simulink model "ForceControl_Quadruped_vmc"  (R2018b)
settings: Solver=FixedStepAuto  StartTime=0.0  StopTime=2  FixedStep=0.001  RelTol=1e-3  EnableMultiTasking=on
undefined symbols (not defined in the file or in its folder): robot, X, Y, Z
libraries: sm_lib x43, nesl_utility x32, Contact_Forces_Lib x4
(part 1 of 3)
settings Model: Creator=gongs  LastModifiedBy=gongs
settings SolverCC: AlgebraicLoopSolver=LineSearch  AutoInsertRateTranBlk=on
settings DataIOCC: LimitDataPoints=on
settings OptimizationCC: LifeSpan=inf
settings DebuggingCC: AllowSymbolicDim=off  SFUnexpectedBacktrackingDiag=warning  SFNoUnconditionalDefaultTransitionDiag=warning  SFExecutionAtInitializationDiag=none
settings SFSimCC: SimUseLocalCustomCode=off
settings RTWCC: RTWUseLocalCustomCode=off
settings CodeAppCC: StateflowObjectComments=on
settings GRTTargetCC: TargetLangStandard=C89/C90 (ANSI)  GeneratePreprocessorConditionals=Disable all
settings ConfigComp: CovMetricSettings=dw  CovHtmlReporting=on  CovSaveCumulativeToWorkspaceVar=on  CovSaveSingleToWorkspaceVar=on  CovExternalEMLEnable=off  CovSFcnEnable=off
settings SimscapeCC: SimscapeNominalValues="[{\"value\":\"10\",\"unit\":\"V\"},{\"value\":\"1\",\"unit\":\"A\"},{\"value\":\"10\",\"unit\":\"N*m\"},{\"value\":\"10\",\"unit\":\"bar\"},{\"value\":\"100\",\"unit\":\"kJ/kg\"},{\"value\":\"1\",\"unit\":\"kW\"},{\"value\":\"300\",\"unit\":\"K\"},{\"value\":\"100\",\"unit\":\"cm^3/s\"},{\"value\":\"1\",\"unit\":\"kN\"},{\"value\":\"1\",\"unit\":\"g/cm^3\"},{\"value\":\"1\",\"unit\":\"l\"},{\"value\":\"1\",\"unit\":\"cm^2\"},{\"value\":\"60\",\"unit\":\"Hz\"}]"  SimscapeLogType=all  SimscapeLogDataHistory=10000
settings ConfigurationSet: Description=SimMechanics 2G
settings DiagnosticsConfigSet: SimMechanicsRigidlyBoundBlock=warning

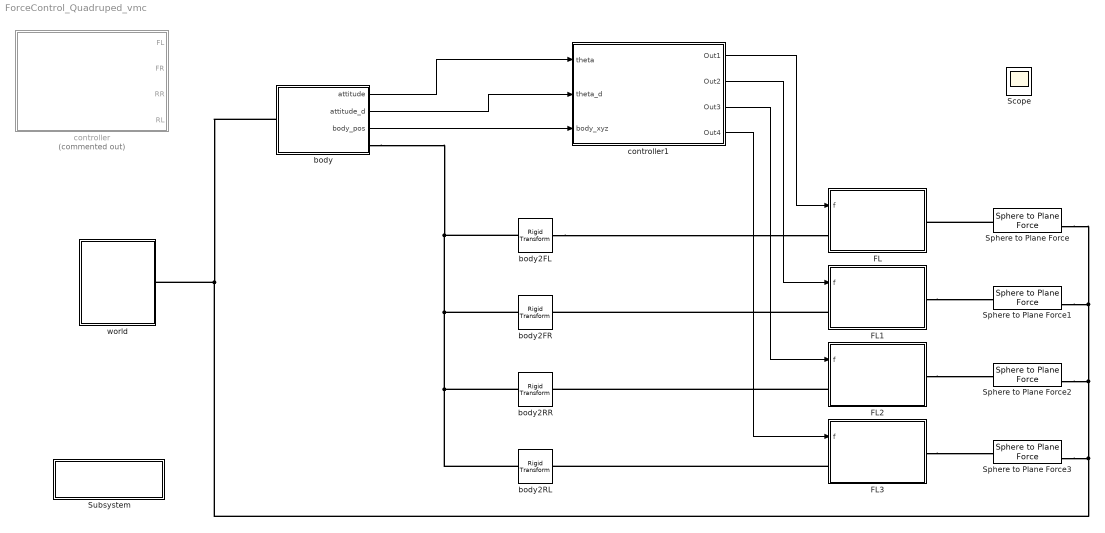
== system ForceControl_Quadruped_vmc ==
  FL : Subsystem
  FL1 : Subsystem
  FL2 : Subsystem
  FL3 : Subsystem
  Sphere to Plane Force{,1..3} (4 alike) : Contact_Forces_Lib/3D/Sphere to Plane Force  sphere_rad=0.05  plane_lenx=5  plane_leny=5  plane_depth=0.05  force_law=Linear  k_contact=1e4  b_contact=1e2  pen_full_damp_F=1e-4  pen_exponent=1  custom_param_1=1  custom_param_2=1  friction_law=Stick-Slip Continuous  mu_kinetic=1  mu_static=5  v_thr=0.001  vis_on=off  vis_opc_en=0  vis_len_plaBz=0.005  vis_clr=[0.9 0.2 0.2]  vis_opc=0.7
  Subsystem : Subsystem
      settings: OpenFcn=open_system('sm_lib')
      mask Display: disp(sprintf('Open Simscape Multibody\nLibrary'));
  body : Subsystem
  body2FL : sm_lib/Frames and Transforms/Rigid Transform  TranslationMethod=Cartesian  TranslationStandardOffset=0.25  TranslationLengthUnit=m  TranslationStandardAxis=+Y  TranslationCartesianOffset=[robot.body.length/2-0.1 robot.body.width/2 0]  TranslationROffset=0  TranslationROffsetUnits=m  TranslationZOffset=0  TranslationZOffsetUnits=m  TranslationThetaOffset=0  TranslationThetaOffsetUnits=deg  RotationMethod=StandardAxis  RotationAngleUnits=deg  RotationStandardAxis=+Y  RotationAngle=90  RotationArbitraryAxis=[0 0 1]  FollAlignAxisA=+X  BaseAlignAxisA=-Z  FollAlignAxisB=+Y  BaseAlignAxisB=+Y  RotationSequenceAxes=FollowerAxes  RotationSequence=XYX  RotationSequenceAngles=[0 0 0]  RotationSequenceAnglesUnits=deg  RotationMatrix=[1 0 0; 0 1 0; 0 0 1]
  body2FR : sm_lib/Frames and Transforms/Rigid Transform  TranslationMethod=Cartesian  TranslationStandardOffset=0.25  TranslationLengthUnit=m  TranslationStandardAxis=+Y  TranslationCartesianOffset=[robot.body.length/2-0.1 -robot.body.width/2 0]  TranslationROffset=0  TranslationROffsetUnits=m  TranslationZOffset=0  TranslationZOffsetUnits=m  TranslationThetaOffset=0  TranslationThetaOffsetUnits=deg  RotationMethod=StandardAxis  RotationAngleUnits=deg  RotationStandardAxis=+Y  RotationAngle=90  RotationArbitraryAxis=[0 0 1]  FollAlignAxisA=+X  BaseAlignAxisA=-Z  FollAlignAxisB=+Y  BaseAlignAxisB=+Y  RotationSequenceAxes=FollowerAxes  RotationSequence=XYX  RotationSequenceAngles=[0 0 0]  RotationSequenceAnglesUnits=deg  RotationMatrix=[1 0 0; 0 1 0; 0 0 1]
  body2RL : sm_lib/Frames and Transforms/Rigid Transform  TranslationMethod=Cartesian  TranslationStandardOffset=0.25  TranslationLengthUnit=m  TranslationStandardAxis=+Y  TranslationCartesianOffset=[-(robot.body.length/2-0.1) robot.body.width/2 0]  TranslationROffset=0  TranslationROffsetUnits=m  TranslationZOffset=0  TranslationZOffsetUnits=m  TranslationThetaOffset=0  TranslationThetaOffsetUnits=deg  RotationMethod=StandardAxis  RotationAngleUnits=deg  RotationStandardAxis=+Y  RotationAngle=90  RotationArbitraryAxis=[0 0 1]  FollAlignAxisA=+X  BaseAlignAxisA=-Z  FollAlignAxisB=+Y  BaseAlignAxisB=+Y  RotationSequenceAxes=FollowerAxes  RotationSequence=XYX  RotationSequenceAngles=[0 0 0]  RotationSequenceAnglesUnits=deg  RotationMatrix=[1 0 0; 0 1 0; 0 0 1]
  body2RR : sm_lib/Frames and Transforms/Rigid Transform  TranslationMethod=Cartesian  TranslationStandardOffset=0.25  TranslationLengthUnit=m  TranslationStandardAxis=+Y  TranslationCartesianOffset=[-(robot.body.length/2-0.1) -robot.body.width/2 0]  TranslationROffset=0  TranslationROffsetUnits=m  TranslationZOffset=0  TranslationZOffsetUnits=m  TranslationThetaOffset=0  TranslationThetaOffsetUnits=deg  RotationMethod=StandardAxis  RotationAngleUnits=deg  RotationStandardAxis=+Y  RotationAngle=90  RotationArbitraryAxis=[0 0 1]  FollAlignAxisA=+X  BaseAlignAxisA=-Z  FollAlignAxisB=+Y  BaseAlignAxisB=+Y  RotationSequenceAxes=FollowerAxes  RotationSequence=XYX  RotationSequenceAngles=[0 0 0]  RotationSequenceAnglesUnits=deg  RotationMatrix=[1 0 0; 0 1 0; 0 0 1]
  controller : Subsystem  Commented=on
  controller1 : Subsystem
  world : Subsystem
  Scope : Scope
  wires:
  body/1(attitude) -> controller1/1(theta)
  body/2(attitude_d) -> controller1/2(theta_d)
  controller1/1(Out1) -> FL/1(f)
  controller1/2(Out2) -> FL1/1(f)
  controller1/3(Out3) -> FL2/1(f)
  controller1/4(Out4) -> FL3/1(f)
  body/3(body_pos) -> controller1/3(body_xyz)
  connections:
  body2FL/RConn1 -- FL/LConn1
  FL1/LConn1 -- body2FR/RConn1
  FL2/LConn1 -- body2RR/RConn1
  FL3/LConn1 -- body2RL/RConn1
  Sphere to Plane Force/LConn1 -- FL/RConn1
  FL1/RConn1 -- Sphere to Plane Force1/LConn1
  FL2/RConn1 -- Sphere to Plane Force2/LConn1
  FL3/RConn1 -- Sphere to Plane Force3/LConn1
  body2RL/LConn1 -- body2RR/LConn1 -- body/RConn1 -- body2FL/LConn1 -- body2FR/LConn1
  Sphere to Plane Force/RConn1 -- body/LConn1 -- world/RConn1 -- Sphere to Plane Force3/RConn1 -- Sphere to Plane Force2/RConn1 -- Sphere to Plane Force1/RConn1

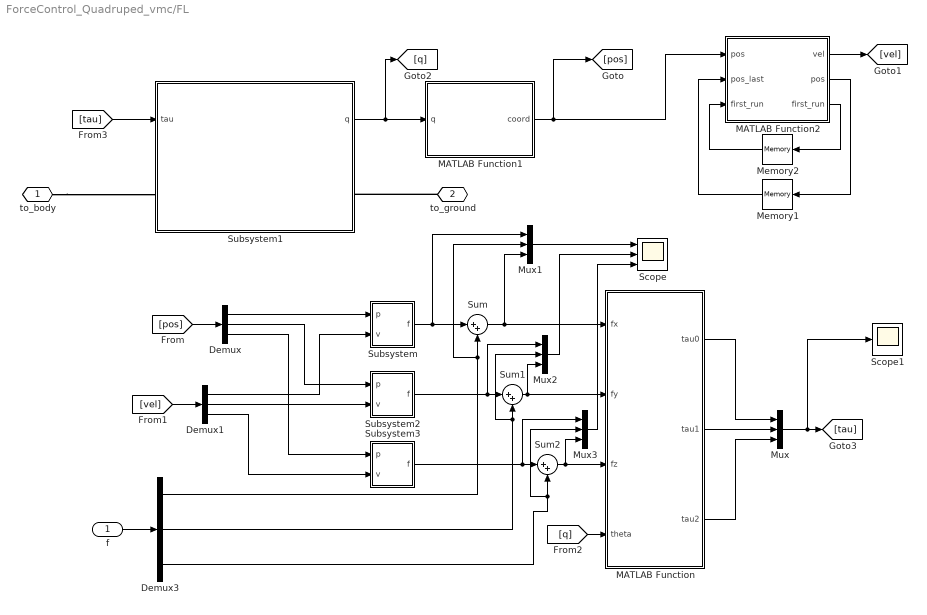
== system ForceControl_Quadruped_vmc/FL ==
  f : Inport
  Demux : Demux  Outputs=3
  Demux1 : Demux  Outputs=3
  Demux3 : Demux  Outputs=3
  MATLAB Function : MATLAB Function  TreatAsAtomicUnit=on
  MATLAB Function1 : MATLAB Function  TreatAsAtomicUnit=on
  MATLAB Function2 : MATLAB Function  TreatAsAtomicUnit=on
  Memory1 : Memory
  Memory2 : Memory  InitialCondition=1
  Mux{,1..3} (4 alike) : Mux  Inputs=3
  Scope : Scope  NumInputPorts=3
  Scope1 : Scope
  Subsystem : Subsystem
  Subsystem1 : Subsystem
  Subsystem2 : Subsystem
  Subsystem3 : Subsystem
  Sum : Sum  Inputs=|++
  Sum1 : Sum  Inputs=|++
  Sum2 : Sum  Inputs=|++
  to_body : PMIOPort  Side=Left
  to_ground : PMIOPort  Port=2  Side=Right
  wires:
  Memory1/1 -> MATLAB Function2/2(pos_last)
  Memory2/1 -> MATLAB Function2/3("first_run ")
  MATLAB Function2/2(pos) -> Memory1/1
  MATLAB Function2/3(first_run) -> Memory2/1
  Subsystem1/1(q) -> MATLAB Function1/1(q), [q]
  MATLAB Function1/1(coord) -> MATLAB Function2/1("pos "), [pos]
  MATLAB Function2/1(vel) -> [vel]
  [q] -> MATLAB Function/4(theta)
  MATLAB Function/1(tau0) -> Mux/1
  MATLAB Function/2(tau1) -> Mux/2
  MATLAB Function/3(tau2) -> Mux/3
  Mux/1 -> Scope1/1, [tau]
  f/1 -> Demux3/1
  [tau] -> Subsystem1/1(tau)
  Subsystem/1(f) -> Mux1/1, Sum/1
  [pos] -> Demux/1
  [vel] -> Demux1/1
  Subsystem2/1(f) -> Mux2/1, Sum1/1
  Subsystem3/1(f) -> Mux3/1, Sum2/1
  Sum/1 -> Mux1/3, MATLAB Function/1(fx)
  Sum1/1 -> Mux2/3, MATLAB Function/2(fy)
  Sum2/1 -> Mux3/3, MATLAB Function/3(fz)
  Demux/1 -> Subsystem/1(p)
  Demux/2 -> Subsystem2/1(p)
  Demux/3 -> Subsystem3/1(p)
  Demux1/1 -> Subsystem/2(v)
  Demux1/2 -> Subsystem2/2(v)
  Demux1/3 -> Subsystem3/2(v)
  Demux3/1 -> Mux1/2, Sum/2
  Demux3/2 -> Mux2/2, Sum1/2
  Demux3/3 -> Mux3/2, Sum2/2
  Mux1/1 -> Scope/1
  Mux2/1 -> Scope/2
  Mux3/1 -> Scope/3
  connections:
  to_body/RConn1 -- Subsystem1/LConn1
  to_ground/RConn1 -- Subsystem1/RConn1

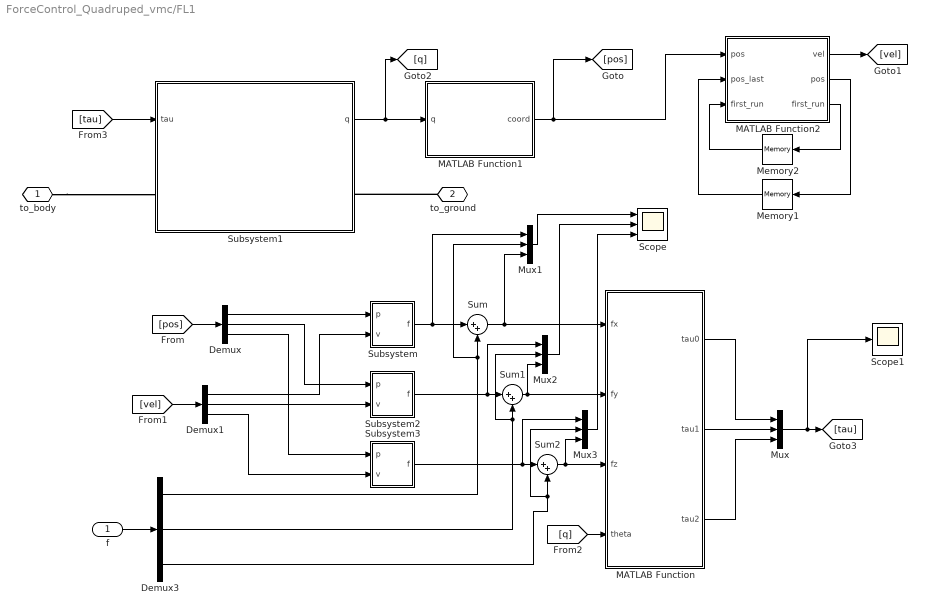
== system ForceControl_Quadruped_vmc/FL1 ==
  f : Inport
  Demux : Demux  Outputs=3
  Demux1 : Demux  Outputs=3
  Demux3 : Demux  Outputs=3
  MATLAB Function : MATLAB Function  TreatAsAtomicUnit=on
  MATLAB Function1 : MATLAB Function  TreatAsAtomicUnit=on
  MATLAB Function2 : MATLAB Function  TreatAsAtomicUnit=on
  Memory1 : Memory
  Memory2 : Memory  InitialCondition=1
  Mux{,1..3} (4 alike) : Mux  Inputs=3
  Scope : Scope  NumInputPorts=3
  Scope1 : Scope
  Subsystem : Subsystem
  Subsystem1 : Subsystem
  Subsystem2 : Subsystem
  Subsystem3 : Subsystem
  Sum : Sum  Inputs=|++
  Sum1 : Sum  Inputs=|++
  Sum2 : Sum  Inputs=|++
  to_body : PMIOPort  Side=Left
  to_ground : PMIOPort  Port=2  Side=Right
  wires:
  Memory1/1 -> MATLAB Function2/2(pos_last)
  Memory2/1 -> MATLAB Function2/3("first_run ")
  MATLAB Function2/2(pos) -> Memory1/1
  MATLAB Function2/3(first_run) -> Memory2/1
  Subsystem1/1(q) -> MATLAB Function1/1(q), [q]
  MATLAB Function1/1(coord) -> MATLAB Function2/1("pos "), [pos]
  MATLAB Function2/1(vel) -> [vel]
  [q] -> MATLAB Function/4(theta)
  MATLAB Function/1(tau0) -> Mux/1
  MATLAB Function/2(tau1) -> Mux/2
  MATLAB Function/3(tau2) -> Mux/3
  Mux/1 -> Scope1/1, [tau]
  f/1 -> Demux3/1
  [tau] -> Subsystem1/1(tau)
  Subsystem/1(f) -> Mux1/1, Sum/1
  [pos] -> Demux/1
  [vel] -> Demux1/1
  Subsystem2/1(f) -> Mux2/1, Sum1/1
  Subsystem3/1(f) -> Mux3/1, Sum2/1
  Sum/1 -> Mux1/3, MATLAB Function/1(fx)
  Sum1/1 -> Mux2/3, MATLAB Function/2(fy)
  Sum2/1 -> Mux3/3, MATLAB Function/3(fz)
  Demux/1 -> Subsystem/1(p)
  Demux/2 -> Subsystem2/1(p)
  Demux/3 -> Subsystem3/1(p)
  Demux1/1 -> Subsystem/2(v)
  Demux1/2 -> Subsystem2/2(v)
  Demux1/3 -> Subsystem3/2(v)
  Demux3/1 -> Mux1/2, Sum/2
  Demux3/2 -> Mux2/2, Sum1/2
  Demux3/3 -> Mux3/2, Sum2/2
  Mux1/1 -> Scope/1
  Mux2/1 -> Scope/2
  Mux3/1 -> Scope/3
  connections:
  to_body/RConn1 -- Subsystem1/LConn1
  to_ground/RConn1 -- Subsystem1/RConn1

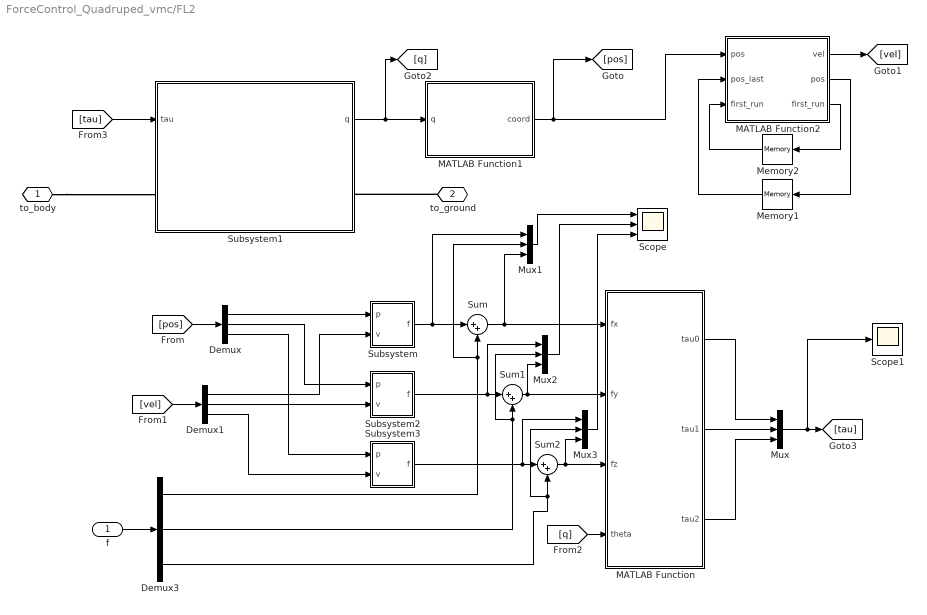
== system ForceControl_Quadruped_vmc/FL2 ==
  f : Inport
  Demux : Demux  Outputs=3
  Demux1 : Demux  Outputs=3
  Demux3 : Demux  Outputs=3
  MATLAB Function : MATLAB Function  TreatAsAtomicUnit=on
  MATLAB Function1 : MATLAB Function  TreatAsAtomicUnit=on
  MATLAB Function2 : MATLAB Function  TreatAsAtomicUnit=on
  Memory1 : Memory
  Memory2 : Memory  InitialCondition=1
  Mux{,1..3} (4 alike) : Mux  Inputs=3
  Scope : Scope  NumInputPorts=3
  Scope1 : Scope
  Subsystem : Subsystem
  Subsystem1 : Subsystem
  Subsystem2 : Subsystem
  Subsystem3 : Subsystem
  Sum : Sum  Inputs=|++
  Sum1 : Sum  Inputs=|++
  Sum2 : Sum  Inputs=|++
  to_body : PMIOPort  Side=Left
  to_ground : PMIOPort  Port=2  Side=Right
  wires:
  Memory1/1 -> MATLAB Function2/2(pos_last)
  Memory2/1 -> MATLAB Function2/3("first_run ")
  MATLAB Function2/2(pos) -> Memory1/1
  MATLAB Function2/3(first_run) -> Memory2/1
  Subsystem1/1(q) -> MATLAB Function1/1(q), [q]
  MATLAB Function1/1(coord) -> MATLAB Function2/1("pos "), [pos]
  MATLAB Function2/1(vel) -> [vel]
  [q] -> MATLAB Function/4(theta)
  MATLAB Function/1(tau0) -> Mux/1
  MATLAB Function/2(tau1) -> Mux/2
  MATLAB Function/3(tau2) -> Mux/3
  Mux/1 -> Scope1/1, [tau]
  f/1 -> Demux3/1
  [tau] -> Subsystem1/1(tau)
  Subsystem/1(f) -> Mux1/1, Sum/1
  [pos] -> Demux/1
  [vel] -> Demux1/1
  Subsystem2/1(f) -> Mux2/1, Sum1/1
  Subsystem3/1(f) -> Mux3/1, Sum2/1
  Sum/1 -> Mux1/3, MATLAB Function/1(fx)
  Sum1/1 -> Mux2/3, MATLAB Function/2(fy)
  Sum2/1 -> Mux3/3, MATLAB Function/3(fz)
  Demux/1 -> Subsystem/1(p)
  Demux/2 -> Subsystem2/1(p)
  Demux/3 -> Subsystem3/1(p)
  Demux1/1 -> Subsystem/2(v)
  Demux1/2 -> Subsystem2/2(v)
  Demux1/3 -> Subsystem3/2(v)
  Demux3/1 -> Mux1/2, Sum/2
  Demux3/2 -> Mux2/2, Sum1/2
  Demux3/3 -> Mux3/2, Sum2/2
  Mux1/1 -> Scope/1
  Mux2/1 -> Scope/2
  Mux3/1 -> Scope/3
  connections:
  to_body/RConn1 -- Subsystem1/LConn1
  to_ground/RConn1 -- Subsystem1/RConn1

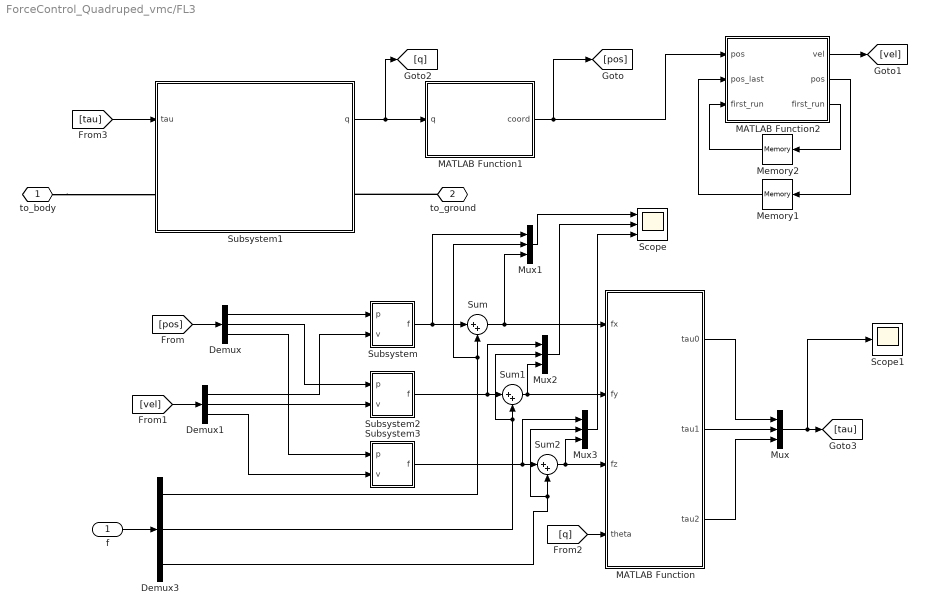
== system ForceControl_Quadruped_vmc/FL3 ==
  f : Inport
  Demux : Demux  Outputs=3
  Demux1 : Demux  Outputs=3
  Demux3 : Demux  Outputs=3
  MATLAB Function : MATLAB Function  TreatAsAtomicUnit=on
  MATLAB Function1 : MATLAB Function  TreatAsAtomicUnit=on
  MATLAB Function2 : MATLAB Function  TreatAsAtomicUnit=on
  Memory1 : Memory
  Memory2 : Memory  InitialCondition=1
  Mux{,1..3} (4 alike) : Mux  Inputs=3
  Scope : Scope  NumInputPorts=3
  Scope1 : Scope
  Subsystem : Subsystem
  Subsystem1 : Subsystem
  Subsystem2 : Subsystem
  Subsystem3 : Subsystem
  Sum : Sum  Inputs=|++
  Sum1 : Sum  Inputs=|++
  Sum2 : Sum  Inputs=|++
  to_body : PMIOPort  Side=Left
  to_ground : PMIOPort  Port=2  Side=Right
  wires:
  Memory1/1 -> MATLAB Function2/2(pos_last)
  Memory2/1 -> MATLAB Function2/3("first_run ")
  MATLAB Function2/2(pos) -> Memory1/1
  MATLAB Function2/3(first_run) -> Memory2/1
  Subsystem1/1(q) -> MATLAB Function1/1(q), [q]
  MATLAB Function1/1(coord) -> MATLAB Function2/1("pos "), [pos]
  MATLAB Function2/1(vel) -> [vel]
  [q] -> MATLAB Function/4(theta)
  MATLAB Function/1(tau0) -> Mux/1
  MATLAB Function/2(tau1) -> Mux/2
  MATLAB Function/3(tau2) -> Mux/3
  Mux/1 -> Scope1/1, [tau]
  f/1 -> Demux3/1
  [tau] -> Subsystem1/1(tau)
  Subsystem/1(f) -> Mux1/1, Sum/1
  [pos] -> Demux/1
  [vel] -> Demux1/1
  Subsystem2/1(f) -> Mux2/1, Sum1/1
  Subsystem3/1(f) -> Mux3/1, Sum2/1
  Sum/1 -> Mux1/3, MATLAB Function/1(fx)
  Sum1/1 -> Mux2/3, MATLAB Function/2(fy)
  Sum2/1 -> Mux3/3, MATLAB Function/3(fz)
  Demux/1 -> Subsystem/1(p)
  Demux/2 -> Subsystem2/1(p)
  Demux/3 -> Subsystem3/1(p)
  Demux1/1 -> Subsystem/2(v)
  Demux1/2 -> Subsystem2/2(v)
  Demux1/3 -> Subsystem3/2(v)
  Demux3/1 -> Mux1/2, Sum/2
  Demux3/2 -> Mux2/2, Sum1/2
  Demux3/3 -> Mux3/2, Sum2/2
  Mux1/1 -> Scope/1
  Mux2/1 -> Scope/2
  Mux3/1 -> Scope/3
  connections:
  to_body/RConn1 -- Subsystem1/LConn1
  to_ground/RConn1 -- Subsystem1/RConn1

== system ForceControl_Quadruped_vmc/Subsystem ==

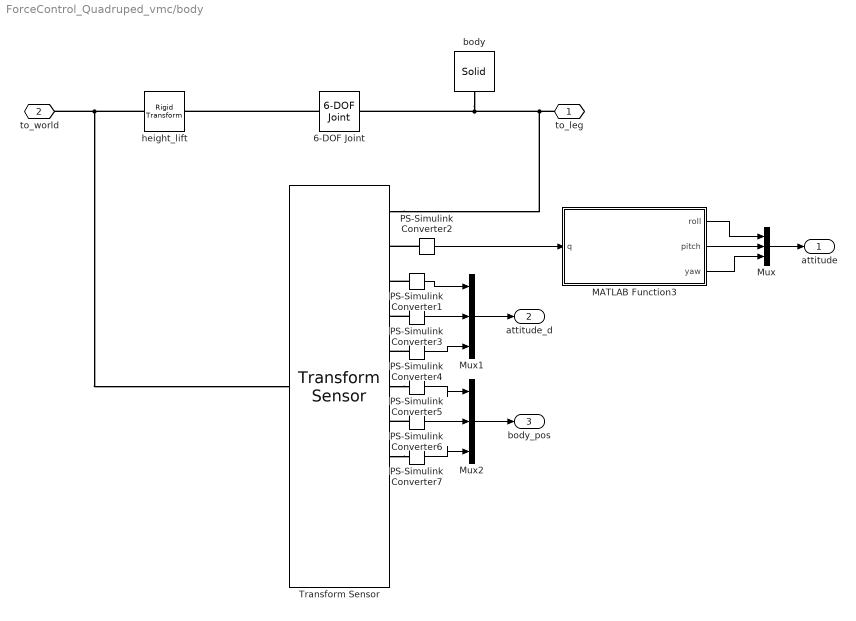
== system ForceControl_Quadruped_vmc/body ==
  6-DOF Joint : sm_lib/Joints/6-DOF Joint  SenseConstraintForce=off  SenseConstraintForceX=off  SenseConstraintForceY=off  SenseConstraintForceZ=off  SenseConstraintTorque=off  SenseConstraintTorqueX=off  SenseConstraintTorqueY=off  SenseConstraintTorqueZ=off  SenseTotalForce=off  SenseTotalForceX=off  SenseTotalForceY=off  SenseTotalForceZ=off  SenseTotalTorque=off  SenseTotalTorqueX=off  SenseTotalTorqueY=off  SenseTotalTorqueZ=off  CompositeWrenchDir=FollowerOnBase  CompositeWrenchFrame=BaseFrame  PxEquilibriumPosition=0  PxEquilibriumPositionUnits=m  PxSpringStiffness=0  PxSpringStiffnessUnits=N/m  PxDampingCoefficient=0  PxDampingCoefficientUnits=N/(m/s)  PxTorqueActuationMode=NoTorque  PxMotionActuationMode=ComputedMotion  PxSensePosition=off  PxSenseVelocity=off  PxSenseAcceleration=off  PxSenseTorqueForce=off  PxPositionTargetSpecify=off  PxPositionTargetPriority=High  PxPositionTargetValue=0  PxPositionTargetValueUnits=m  PxVelocityTargetSpecify=off  PxVelocityTargetPriority=High  PxVelocityTargetValue=0  PxVelocityTargetValueUnits=m/s  PyEquilibriumPosition=0  PyEquilibriumPositionUnits=m  PySpringStiffness=0  PySpringStiffnessUnits=N/m  PyDampingCoefficient=0  PyDampingCoefficientUnits=N/(m/s)  PyTorqueActuationMode=NoTorque  PyMotionActuationMode=ComputedMotion  PySensePosition=off  PySenseVelocity=off  PySenseAcceleration=off  PySenseTorqueForce=off  PyPositionTargetSpecify=off  PyPositionTargetPriority=High  PyPositionTargetValue=0  PyPositionTargetValueUnits=m  PyVelocityTargetSpecify=off  PyVelocityTargetPriority=High  PyVelocityTargetValue=0  PyVelocityTargetValueUnits=m/s  PzEquilibriumPosition=0  PzEquilibriumPositionUnits=m  PzSpringStiffness=0  PzSpringStiffnessUnits=N/m  PzDampingCoefficient=0  PzDampingCoefficientUnits=N/(m/s)  PzTorqueActuationMode=NoTorque  PzMotionActuationMode=ComputedMotion  PzSensePosition=off  PzSenseVelocity=off  PzSenseAcceleration=off  PzSenseTorqueForce=off  PzPositionTargetSpecify=off  PzPositionTargetPriority=High  PzPositionTargetValue=0  PzPositionTargetValueUnits=m  PzVelocityTargetSpecify=off  PzVelocityTargetPriority=High  PzVelocityTargetValue=0  PzVelocityTargetValueUnits=m/s  SphDefPosRotationMethod=None  SphDefPosRotationAngleUnits=deg  SphDefPosRotationStandardAxis=+Z  SphDefPosRotationAngle=0.0  SphDefPosRotationArbitraryAxis=[0 0 1]  SphDefPosFollAlignAxisA=+X  SphDefPosBaseAlignAxisA=+Y  SphDefPosFollAlignAxisB=+Y  SphDefPosBaseAlignAxisB=+Z  SphDefPosRotationSequenceAxes=FollowerAxes  SphDefPosRotationSequence=XYX  SphDefPosRotationSequenceAngles=[0 0 0]  SphDefPosRotationSequenceAnglesUnits=deg  SphDefPosRotationMatrix=[1 0 0; 0 1 0; 0 0 1]  SphEqPosRotationMethod=None  SphEqPosRotationAngleUnits=deg  SphEqPosRotationStandardAxis=+Z  SphEqPosRotationAngle=0.0  SphEqPosRotationArbitraryAxis=[0 0 1]  SphEqPosFollAlignAxisA=+X  SphEqPosBaseAlignAxisA=+Y  SphEqPosFollAlignAxisB=+Y  SphEqPosBaseAlignAxisB=+Z  SphEqPosRotationSequenceAxes=FollowerAxes  SphEqPosRotationSequence=XYX  SphEqPosRotationSequenceAngles=[0 0 0]  SphEqPosRotationSequenceAnglesUnits=deg  SphEqPosRotationMatrix=[1 0 0; 0 1 0; 0 0 1]  SphSpringStiffness=0  SphSpringStiffnessUnits=N*m/deg  SphDampingCoefficient=0  SphDampingCoefficientUnits=N*m/(deg/s)  SphActuateTorqueX=off  SphActuateTorqueY=off  SphActuateTorqueZ=off  SphActuateTorque=off  SphTorqueActuationMode=NoTorque  SphMotionActuationMode=ComputedMotion  SphActuationFrame=BaseFrame  SphSensePosition=off  SphSenseVelocityX=off  SphSenseVelocityY=off  SphSenseVelocityZ=off  SphSenseVelocity=off  SphSenseAccelerationX=off  SphSenseAccelerationY=off  SphSenseAccelerationZ=off  SphSenseAcceleration=off  SphSenseTorqueX=off  SphSenseTorqueY=off  SphSenseTorqueZ=off  SphSenseTorqueForce=off  SphSensingFrame=BaseFrame  SphPositionTargetRotationMethod=None  SphPositionTargetRotationAngleUnits=deg  SphPositionTargetRotationStandardAxis=+Z  SphPositionTargetRotationAngle=0.0  SphPositionTargetRotationArbitraryAxis=[0 0 1]  SphPositionTargetFollAlignAxisA=+X  SphPositionTargetBaseAlignAxisA=+Y  SphPositionTargetFollAlignAxisB=+Y  SphPositionTargetBaseAlignAxisB=+Z  SphPositionTargetRotationSequenceAxes=FollowerAxes  SphPositionTargetRotationSequence=XYX  SphPositionTargetRotationSequenceAngles=[0 0 0]  SphPositionTargetRotationSequenceAnglesUnits=deg  SphPositionTargetRotationMatrix=[1 0 0; 0 1 0; 0 0 1]  SphPositionTargetSpecify=off  SphPositionTargetPriority=High  SphVelocityTargetValue=[0 0 0]  SphVelocityTargetValueUnits=deg/s  SphVelocityTargetSpecify=off  SphVelocityTargetPriority=High  SphVelocityTargetInFollowerFrame=on
  MATLAB Function3 : MATLAB Function  TreatAsAtomicUnit=on
  Mux : Mux  Inputs=3
  Mux1 : Mux  Inputs=3
  Mux2 : Mux  Inputs=3
  PS-Simulink Converter{1..7} (7 alike) : nesl_utility/PS-Simulink Converter  PhysicalDomain=network_engine_domain  SubClassName=ps_output  LeftPortType=input  RightPortType=output  PseudoPeriodic=off  Frequencies=[]  Unit=1  AffineConversion=off
  Transform Sensor : sm_lib/Frames and Transforms/Transform Sensor  MeasurementFrame=World  SenseAngle=off  SenseAxis=off  SenseAngle1=off  SenseAngle2=off  SenseAngle3=off  SenseQ=on  SenseR=off  SenseOmegaX=on  SenseOmegaY=on  SenseOmegaZ=on  SenseOmega1=off  SenseOmega2=off  SenseOmega3=off  SenseQDot=off  SenseRDot=off  SenseAlphaX=off  SenseAlphaY=off  SenseAlphaZ=off  SenseAlpha1=off  SenseAlpha2=off  SenseAlpha3=off  SenseQDDot=off  SenseRDDot=off  SenseX=on  SenseY=on  SenseZ=on  SenseRad=off  SenseAzim=off  SenseDist=off  SenseInc=off  SenseXDot=on  SenseYDot=on  SenseZDot=on  SenseRadDot=off  SenseAzimDot=off  SenseDistDot=off  SenseIncDot=off  SenseXDDot=off  SenseYDDot=off  SenseZDDot=off  SenseRadDDot=off  SenseAzimDDot=off  SenseDistDDot=off  SenseIncDDot=off
  body : sm_lib/Body Elements/Solid  InertiaType=CalculateFromGeometry  Mass=robot.body.weight  MassUnits=kg  CenterOfMass=[0 0 0]  CenterOfMassUnits=m  MomentsOfInertia=[1 1 1]  MomentsOfInertiaUnits=kg*m^2  ProductsOfInertia=[0 0 0]  ProductsOfInertiaUnits=kg*m^2  BasedOnType=Mass  Density=1000  DensityUnits=kg/m^3  DoExposeReferenceFrame=on  SerializedFrames=<Frames/>  GraphicType=FromGeometry  MarkerShape=Sphere  MarkerSize=10  GraphicVisPropType=SimpleVisualProperties  GraphicDiffuseColor=[1.0 0.6 0.2]  GraphicSpecularColor=[0.5 0.5 0.5 1.0]  GraphicAmbientColor=[0.15 0.15 0.15 1.0]  GraphicEmissiveColor=[0.0 0.0 0.0 1.0]  GraphicShininess=75  GraphicOpacity=1.0  GeometryShape=Brick  RectangleSize=[1 1]  RectangleSizeUnits=m  BrickDimensions=[robot.body.length robot.body.width robot.body.thickness]  BrickDimensionUnits=m  CylinderRadius=1  CylinderRadiusUnits=m  CylinderLength=1  CylinderLengthUnits=m  SphereRadius=1  SphereRadiusUnits=m  EllipsoidRadii=[1 1 1]  EllipsoidRadiiUnits=m  ExtrusionCrossSection=[1 1; -1 1; -1 -1; 1 -1]  ExtrusionCrossSectionUnits=m  ExtrusionLength=1  ExtrusionLengthUnits=m  PolygonNumSides=3  PolygonOuterRadius=1  PolygonOuterRadiusUnits=m  ExtGeomFileType=STEP  ExtGeomFileUnits=m  RevolutionCrossSection=[1 1; 1 -1; 2 -1; 2 1]  RevolutionCrossSectionUnits=m  RevolutionExtent=Full  RevolutionAngle=180  RevolutionAngleUnits=deg
  height_lift : sm_lib/Frames and Transforms/Rigid Transform  TranslationMethod=Cartesian  TranslationStandardOffset=1.5  TranslationLengthUnit=m  TranslationStandardAxis=+Z  TranslationCartesianOffset=[0 0 0.9]  TranslationROffset=0  TranslationROffsetUnits=m  TranslationZOffset=0  TranslationZOffsetUnits=m  TranslationThetaOffset=0  TranslationThetaOffsetUnits=deg  RotationMethod=None  RotationAngleUnits=deg  RotationStandardAxis=+Z  RotationAngle=0.0  RotationArbitraryAxis=[0 0 1]  FollAlignAxisA=+X  BaseAlignAxisA=+Y  FollAlignAxisB=+Y  BaseAlignAxisB=+Z  RotationSequenceAxes=FollowerAxes  RotationSequence=XYX  RotationSequenceAngles=[0 0 0]  RotationSequenceAnglesUnits=deg  RotationMatrix=[1 0 0; 0 1 0; 0 0 1]
  to_leg : PMIOPort  Side=Right
  to_world : PMIOPort  Port=2  Side=Left
  attitude : Outport
  attitude_d : Outport  Port=2
  body_pos : Outport  Port=3
  wires:
  PS-Simulink Converter2/1 -> MATLAB Function3/1(q)
  MATLAB Function3/1(roll) -> Mux/1
  MATLAB Function3/2(pitch) -> Mux/2
  MATLAB Function3/3(yaw) -> Mux/3
  PS-Simulink Converter3/1 -> Mux1/2
  PS-Simulink Converter1/1 -> Mux1/1
  PS-Simulink Converter4/1 -> Mux1/3
  Mux/1 -> attitude/1
  Mux1/1 -> attitude_d/1
  PS-Simulink Converter5/1 -> Mux2/1
  PS-Simulink Converter6/1 -> Mux2/2
  PS-Simulink Converter7/1 -> Mux2/3
  Mux2/1 -> body_pos/1
  connections:
  6-DOF Joint/LConn1 -- height_lift/RConn1
  PS-Simulink Converter2/LConn1 -- Transform Sensor/RConn2
  to_leg/RConn1 -- 6-DOF Joint/RConn1 -- body/RConn1 -- Transform Sensor/RConn1
  PS-Simulink Converter1/LConn1 -- Transform Sensor/RConn3
  PS-Simulink Converter3/LConn1 -- Transform Sensor/RConn4
  PS-Simulink Converter4/LConn1 -- Transform Sensor/RConn5
  PS-Simulink Converter6/LConn1 -- Transform Sensor/RConn7
  Transform Sensor/RConn6 -- PS-Simulink Converter5/LConn1
  Transform Sensor/RConn8 -- PS-Simulink Converter7/LConn1
  height_lift/LConn1 -- Transform Sensor/LConn1 -- to_world/RConn1

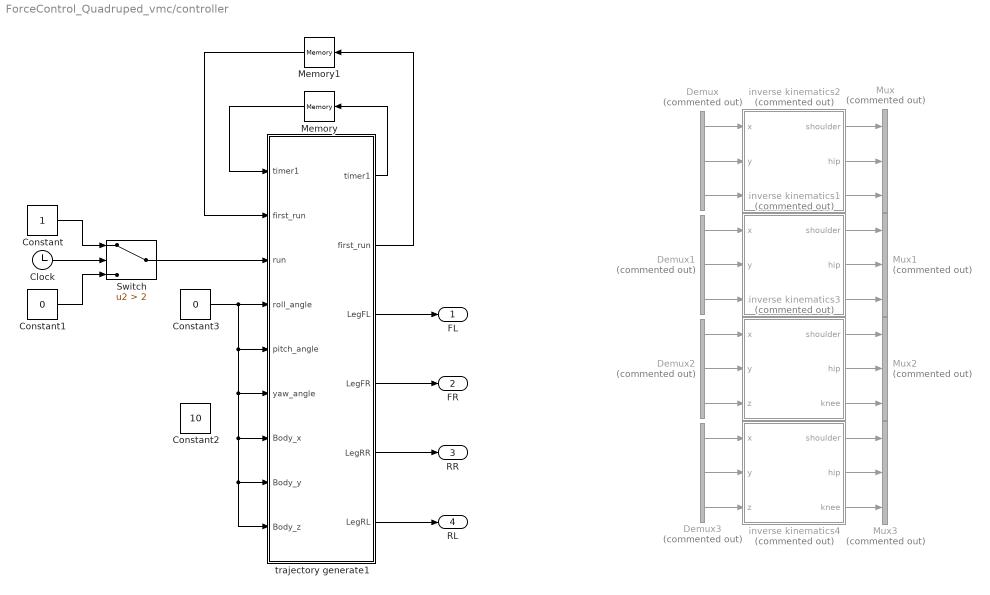
== system ForceControl_Quadruped_vmc/controller ==
  Clock : Clock
  Constant : Constant
  Constant1 : Constant  Value=0
  Constant2 : Constant  Value=10
  Constant3 : Constant  Value=0
  Demux{,1..3} (4 alike) : Demux  Commented=on  Outputs=3
  Memory : Memory
  Memory1 : Memory  InitialCondition=1
  Mux{,1..3} (4 alike) : Mux  Commented=on  Inputs=3
  Switch : Switch  Criteria=u2 > Threshold  Threshold=2
  inverse kinematics1 : MATLAB Function  Commented=on  TreatAsAtomicUnit=on
  inverse kinematics2 : MATLAB Function  Commented=on  TreatAsAtomicUnit=on
  inverse kinematics3 : MATLAB Function  Commented=on  TreatAsAtomicUnit=on
  inverse kinematics4 : MATLAB Function  Commented=on  TreatAsAtomicUnit=on
  trajectory generate1 : MATLAB Function  TreatAsAtomicUnit=on
  FL : Outport
  FR : Outport  Port=2
  "RR " : Outport  Port=3
  RL : Outport  Port=4
  wires:
  trajectory generate1/3(LegFL) -> FL/1
  trajectory generate1/4(LegFR) -> FR/1
  trajectory generate1/5(LegRR) -> "RR "/1
  trajectory generate1/6(LegRL) -> RL/1
  trajectory generate1/1(timer1) -> Memory/1
  Memory/1 -> trajectory generate1/1("timer1 ")
  Switch/1 -> trajectory generate1/3(run)
  Clock/1 -> Switch/2
  Constant/1 -> Switch/1
  Constant1/1 -> Switch/3
  trajectory generate1/2(first_run) -> Memory1/1
  Memory1/1 -> trajectory generate1/2("first_run ")
  Constant3/1 -> trajectory generate1/4(roll_angle), trajectory generate1/5(pitch_angle), trajectory generate1/6(yaw_angle), trajectory generate1/7(Body_x), trajectory generate1/8(Body_y), trajectory generate1/9(Body_z)
  Demux1/3 -> inverse kinematics1/3(z)
  inverse kinematics4/3(knee) -> Mux3/3
  Demux2/3 -> inverse kinematics3/3(z)
  inverse kinematics4/2(hip) -> Mux3/2
  Demux/3 -> inverse kinematics2/3(z)
  inverse kinematics1/1(shoulder) -> Mux1/1
  inverse kinematics3/2(hip) -> Mux2/2
  Demux/2 -> inverse kinematics2/2(y)
  Demux3/3 -> inverse kinematics4/3(z)
  inverse kinematics1/3(knee) -> Mux1/3
  inverse kinematics3/3(knee) -> Mux2/3
  Demux/1 -> inverse kinematics2/1(x)
  Demux3/2 -> inverse kinematics4/2(y)
  inverse kinematics4/1(shoulder) -> Mux3/1
  inverse kinematics2/3(knee) -> Mux/3
  Demux2/1 -> inverse kinematics3/1(x)
  inverse kinematics2/1(shoulder) -> Mux/1
  inverse kinematics2/2(hip) -> Mux/2
  inverse kinematics1/2(hip) -> Mux1/2
  inverse kinematics3/1(shoulder) -> Mux2/1
  Demux3/1 -> inverse kinematics4/1(x)
  Demux1/1 -> inverse kinematics1/1(x)
  Demux2/2 -> inverse kinematics3/2(y)
  Demux1/2 -> inverse kinematics1/2(y)

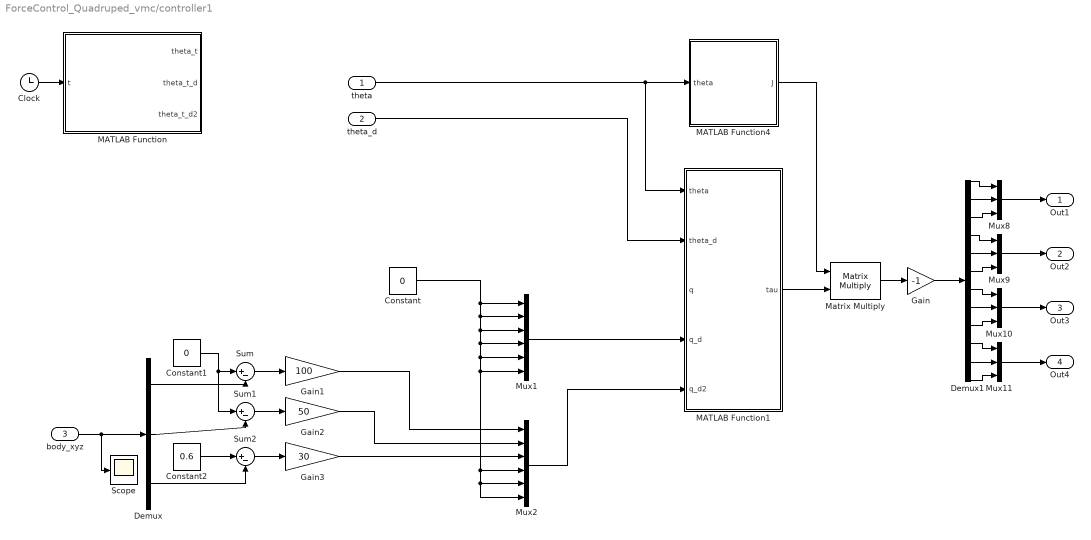
== system ForceControl_Quadruped_vmc/controller1 ==
  theta : Inport
  theta_d : Inport  Port=2
  body_xyz : Inport  Port=3
  Clock : Clock
  Constant : Constant  Value=0
  Constant1 : Constant  Value=0
  Constant2 : Constant  Value=0.6
  Demux : Demux  Outputs=3
  Demux1 : Demux  Outputs=12
  Gain : Gain  Gain=-1
  Gain1 : Gain  Gain=100
  Gain2 : Gain  Gain=50
  Gain3 : Gain  Gain=30
  MATLAB Function : MATLAB Function  TreatAsAtomicUnit=on
  MATLAB Function1 : MATLAB Function  TreatAsAtomicUnit=on
  MATLAB Function4 : MATLAB Function  TreatAsAtomicUnit=on
  Matrix Multiply : Product  Multiplication=Matrix(*)
  Mux1 : Mux  Inputs=6
  Mux{8..11} (4 alike) : Mux  Inputs=3
  Mux2 : Mux  Inputs=6
  Scope : Scope
  Sum : Sum  Inputs=|+-
  Sum1 : Sum  Inputs=|+-
  Sum2 : Sum  Inputs=|+-
  Out1 : Outport
  Out2 : Outport  Port=2
  Out3 : Outport  Port=3
  Out4 : Outport  Port=4
  wires:
  MATLAB Function4/1(J) -> Matrix Multiply/1
  Matrix Multiply/1 -> Gain/1
  Demux1/8 -> Mux10/2
  Demux1/7 -> Mux10/1
  theta/1 -> MATLAB Function1/1(theta), MATLAB Function4/1(theta)
  Demux1/2 -> Mux8/2
  theta_d/1 -> MATLAB Function1/2(theta_d)
  MATLAB Function1/1(tau) -> Matrix Multiply/2
  Constant/1 -> Mux1/1, Mux1/2, Mux1/3, Mux1/4, Mux1/5, Mux1/6, Mux2/4, Mux2/5, Mux2/6
  Clock/1 -> MATLAB Function/1(t)
  Mux1/1 -> MATLAB Function1/4(q_d)
  Mux2/1 -> MATLAB Function1/5(q_d2)
  Demux1/9 -> Mux10/3
  Demux1/3 -> Mux8/3
  Demux1/6 -> Mux9/3
  Demux1/5 -> Mux9/2
  Demux1/10 -> Mux11/1
  Demux1/12 -> Mux11/3
  Demux1/11 -> Mux11/2
  Demux1/4 -> Mux9/1
  Demux1/1 -> Mux8/1
  Mux8/1 -> Out1/1
  Mux9/1 -> Out2/1
  Mux11/1 -> Out4/1
  Mux10/1 -> Out3/1
  Gain/1 -> Demux1/1
  body_xyz/1 -> Scope/1, Demux/1
  Sum/1 -> Gain1/1
  Sum1/1 -> Gain2/1
  Sum2/1 -> Gain3/1
  Demux/1 -> Sum/2
  Demux/2 -> Sum1/2
  Demux/3 -> Sum2/2
  Constant1/1 -> Sum1/1, Sum/1
  Constant2/1 -> Sum2/1
  Gain1/1 -> Mux2/1
  Gain2/1 -> Mux2/2
  Gain3/1 -> Mux2/3

== system ForceControl_Quadruped_vmc/world ==
  Mechanism Configuration : sm_lib/Utilities/Mechanism Configuration  UniformGravity=Constant  GravityVector=[0 0 -9.80665]  GravityUnits=m/s^2  LinearizationDelta=0.001
  Solver Configuration : nesl_utility/Solver Configuration  PhysicalDomain=network_engine_domain  SubClassName=solver  LeftPortType=input  RightPortType=generic  Tones=[]  Harmonics=[]  SimulateNoise=off  Profile=off  UseLocalSampling=off  EnableSwitchedLinearOptims=on  FrequencyDomain=off  UseCCode=off  RelTol=0.001  AbsTol=1e-06  MinStep=1e-09  ToWorkspace=off  RevertToSquareIcSolve=off  NumHomotopyIterations=100  PhasorMode=off  PhasorModeNumHarmonics=1  DoDC=off  ResidualTolerance=1e-09  UseLocalSolver=off  LocalSolverChoice=NE_BACKWARD_EULER_ADVANCER  LocalSolverSampleTime=0.001  DoFixedCost=off  MaxNonlinIter=3  MaxModeIter=2  LinearAlgebra=Sparse  EquationFormulation=NE_TIME_EF  DelaysMemoryBudget=1024  AutomaticFiltering=on  FilteringTimeConstant=0.001  PartitionStorageMethod=AS_NEEDED  PartitionMemoryBudget=1024
  World Frame : sm_lib/Frames and Transforms/World Frame
  floor : sm_lib/Body Elements/Solid  InertiaType=CalculateFromGeometry  Mass=1  MassUnits=kg  CenterOfMass=[0 0 0]  CenterOfMassUnits=m  MomentsOfInertia=[1 1 1]  MomentsOfInertiaUnits=kg*m^2  ProductsOfInertia=[0 0 0]  ProductsOfInertiaUnits=kg*m^2  BasedOnType=Density  Density=1000  DensityUnits=kg/m^3  DoExposeReferenceFrame=on  SerializedFrames=<Frames/>  GraphicType=FromGeometry  MarkerShape=Sphere  MarkerSize=10  GraphicVisPropType=SimpleVisualProperties  GraphicDiffuseColor=[0.5 0.5 0.5]  GraphicSpecularColor=[0.5 0.5 0.5 1.0]  GraphicAmbientColor=[0.15 0.15 0.15 1.0]  GraphicEmissiveColor=[0.0 0.0 0.0 1.0]  GraphicShininess=75  GraphicOpacity=1.0  GeometryShape=Brick  RectangleSize=[1 1]  RectangleSizeUnits=m  BrickDimensions=[5 5 0.1]  BrickDimensionUnits=m  CylinderRadius=1  CylinderRadiusUnits=m  CylinderLength=1  CylinderLengthUnits=m  SphereRadius=1  SphereRadiusUnits=m  EllipsoidRadii=[1 1 1]  EllipsoidRadiiUnits=m  ExtrusionCrossSection=[1 1; -1 1; -1 -1; 1 -1]  ExtrusionCrossSectionUnits=m  ExtrusionLength=1  ExtrusionLengthUnits=m  PolygonNumSides=3  PolygonOuterRadius=1  PolygonOuterRadiusUnits=m  ExtGeomFileType=STEP  ExtGeomFileUnits=m  RevolutionCrossSection=[1 1; 1 -1; 2 -1; 2 1]  RevolutionCrossSectionUnits=m  RevolutionExtent=Full  RevolutionAngle=180  RevolutionAngleUnits=deg
  to_body : PMIOPort  Side=Right
  connections:
  World Frame/RConn1 -- to_body/RConn1 -- floor/RConn1 -- Mechanism Configuration/RConn1 -- Solver Configuration/RConn1

== system ForceControl_Quadruped_vmc/FL/Subsystem ==
  p : Inport
  v : Inport  Port=2
  Constant : Constant  Value=0
  Constant1 : Constant  Value=0
  Gain : Gain  Gain=10
  Gain1 : Gain
  Sum : Sum  Inputs=|+-
  Sum1 : Sum  Inputs=|+-
  Sum2 : Sum  Inputs=|++
  f : Outport
  wires:
  Sum1/1 -> Gain1/1
  Constant1/1 -> Sum1/1
  Sum/1 -> Gain/1
  Constant/1 -> Sum/1
  Gain1/1 -> Sum2/2
  Gain/1 -> Sum2/1
  v/1 -> Sum1/2
  Sum2/1 -> f/1
  p/1 -> Sum/2

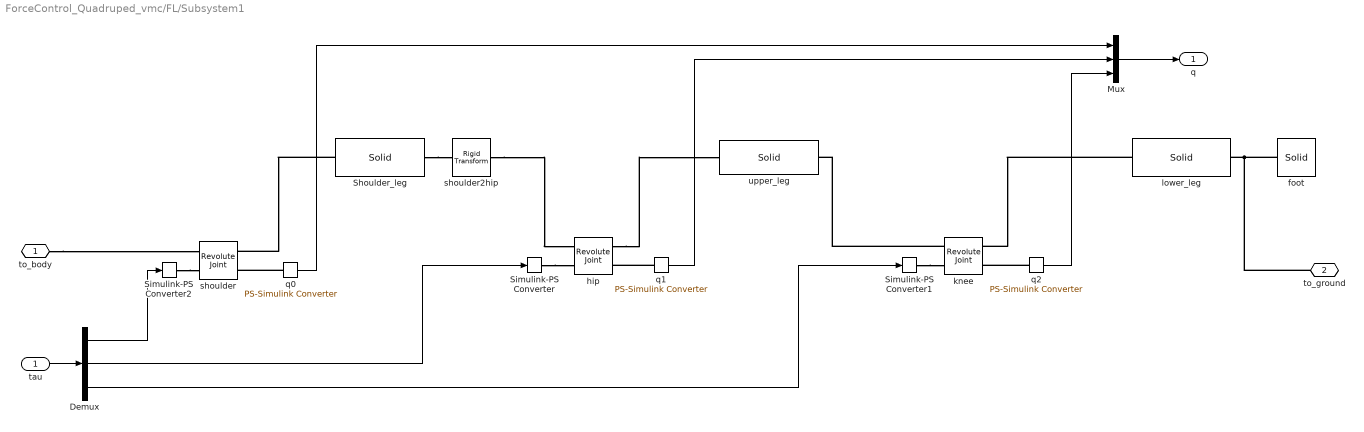
== system ForceControl_Quadruped_vmc/FL/Subsystem1 ==
  tau : Inport
  Demux : Demux  Outputs=3
  Mux : Mux  Inputs=3
  Shoulder_leg : sm_lib/Body Elements/Solid  InertiaType=CalculateFromGeometry  Mass=0  MassUnits=kg  CenterOfMass=[0 0 0]  CenterOfMassUnits=m  MomentsOfInertia=[1 1 1]  MomentsOfInertiaUnits=kg*m^2  ProductsOfInertia=[0 0 0]  ProductsOfInertiaUnits=kg*m^2  BasedOnType=Mass  Density=1000  DensityUnits=kg/m^3  DoExposeReferenceFrame=off  SerializedFrames=<Frames><Frame><Id>Frame1</Id><Value><Name>to_shoulder</Name><Origin><Source>ReferenceFrame</Source><FeatureName></FeatureName></Origin><PrimaryAxis><DefinedDirection>+Z</DefinedDirection><Source>ReferenceFrame</Source><SourceDirection>+Z</SourceDirection><FeatureName></FeatureName></PrimaryAxis><SecondaryAxis><DefinedDirection>+X</DefinedDirection><Source>ReferenceFrame</Source><SourceDirection>+X</SourceDirection><FeatureName></FeatureName></SecondaryAxis></Value></Frame><Frame><Id>Frame2</Id><Value><Name>to_hip</Name><Origin><Source>ReferenceFrame</Source><FeatureName></FeatureName></Origin><PrimaryAxis><DefinedDirection>+Z</DefinedDirection><Source>ReferenceFrame</Source><SourceDirection>+Z</SourceDirection><FeatureName></FeatureName></PrimaryAxis><SecondaryAxis><DefinedDirection>+X</DefinedDirection><Source>ReferenceFrame</Source><SourceDirection>+X</SourceDirection><FeatureName></FeatureName></SecondaryAxis></Value></Frame></Frames>  GraphicType=FromGeometry  MarkerShape=Sphere  MarkerSize=10  GraphicVisPropType=SimpleVisualProperties  GraphicDiffuseColor=[1.0 0.0 0.2]  GraphicSpecularColor=[0.5 0.5 0.5 1.0]  GraphicAmbientColor=[0.15 0.15 0.15 1.0]  GraphicEmissiveColor=[0.0 0.0 0.0 1.0]  GraphicShininess=75  GraphicOpacity=1.0  GeometryShape=Brick  RectangleSize=[1 1]  RectangleSizeUnits=m  BrickDimensions=[0.06 0.06 0.06]  BrickDimensionUnits=m  CylinderRadius=1  CylinderRadiusUnits=m  CylinderLength=1  CylinderLengthUnits=m  SphereRadius=1  SphereRadiusUnits=m  EllipsoidRadii=[1 1 1]  EllipsoidRadiiUnits=m  ExtrusionCrossSection=[1 1; -1 1; -1 -1; 1 -1]  ExtrusionCrossSectionUnits=m  ExtrusionLength=1  ExtrusionLengthUnits=m  PolygonNumSides=3  PolygonOuterRadius=1  PolygonOuterRadiusUnits=m  ExtGeomFileType=STEP  ExtGeomFileUnits=m  RevolutionCrossSection=[1 1; 1 -1; 2 -1; 2 1]  RevolutionCrossSectionUnits=m  RevolutionExtent=Full  RevolutionAngle=180  RevolutionAngleUnits=deg
  Simulink-PS Converter : nesl_utility/Simulink-PS Converter  PhysicalDomain=network_engine_domain  SubClassName=ps_input  LeftPortType=input  RightPortType=output  PseudoPeriodic=off  Frequencies=[]  NoiseDistribution=none  NoiseParameters=[]  Unit=1  AffineConversion=off  FilteringAndDerivatives=filter  SimscapeFilterOrder=2  InputFilterTimeConstant=0.001  UdotUserProvided=0
  Simulink-PS Converter1 : nesl_utility/Simulink-PS Converter  PhysicalDomain=network_engine_domain  SubClassName=ps_input  LeftPortType=input  RightPortType=output  PseudoPeriodic=off  Frequencies=[]  NoiseDistribution=none  NoiseParameters=[]  Unit=1  AffineConversion=off  FilteringAndDerivatives=filter  SimscapeFilterOrder=2  InputFilterTimeConstant=0.001  UdotUserProvided=0
  Simulink-PS Converter2 : nesl_utility/Simulink-PS Converter  PhysicalDomain=network_engine_domain  SubClassName=ps_input  LeftPortType=input  RightPortType=output  PseudoPeriodic=off  Frequencies=[]  NoiseDistribution=none  NoiseParameters=[]  Unit=1  AffineConversion=off  FilteringAndDerivatives=filter  SimscapeFilterOrder=2  InputFilterTimeConstant=0.001  UdotUserProvided=0
  foot : sm_lib/Body Elements/Solid  InertiaType=CalculateFromGeometry  Mass=0  MassUnits=kg  CenterOfMass=[0 0 0]  CenterOfMassUnits=m  MomentsOfInertia=[1 1 1]  MomentsOfInertiaUnits=kg*m^2  ProductsOfInertia=[0 0 0]  ProductsOfInertiaUnits=kg*m^2  BasedOnType=Mass  Density=1000  DensityUnits=kg/m^3  DoExposeReferenceFrame=on  SerializedFrames=<Frames/>  GraphicType=FromGeometry  MarkerShape=Sphere  MarkerSize=10  GraphicVisPropType=SimpleVisualProperties  GraphicDiffuseColor=[1.0 0.2 0.2]  GraphicSpecularColor=[0.5 0.5 0.5 1.0]  GraphicAmbientColor=[0.15 0.15 0.15 1.0]  GraphicEmissiveColor=[0.0 0.0 0.0 1.0]  GraphicShininess=75  GraphicOpacity=1.0  GeometryShape=Sphere  RectangleSize=[1 1]  RectangleSizeUnits=m  BrickDimensions=[1 1 1]  BrickDimensionUnits=m  CylinderRadius=1  CylinderRadiusUnits=m  CylinderLength=1  CylinderLengthUnits=m  SphereRadius=0.05  SphereRadiusUnits=m  EllipsoidRadii=[1 1 1]  EllipsoidRadiiUnits=m  ExtrusionCrossSection=[1 1; -1 1; -1 -1; 1 -1]  ExtrusionCrossSectionUnits=m  ExtrusionLength=1  ExtrusionLengthUnits=m  PolygonNumSides=3  PolygonOuterRadius=1  PolygonOuterRadiusUnits=m  ExtGeomFileType=STEP  ExtGeomFileUnits=m  RevolutionCrossSection=[1 1; 1 -1; 2 -1; 2 1]  RevolutionCrossSectionUnits=m  RevolutionExtent=Full  RevolutionAngle=180  RevolutionAngleUnits=deg
  hip : sm_lib/Joints/Revolute Joint  SenseConstraintForce=off  SenseConstraintForceX=off  SenseConstraintForceY=off  SenseConstraintForceZ=off  SenseConstraintTorque=off  SenseConstraintTorqueX=off  SenseConstraintTorqueY=off  SenseConstraintTorqueZ=off  SenseTotalForce=off  SenseTotalForceX=off  SenseTotalForceY=off  SenseTotalForceZ=off  SenseTotalTorque=off  SenseTotalTorqueX=off  SenseTotalTorqueY=off  SenseTotalTorqueZ=off  CompositeWrenchDir=FollowerOnBase  CompositeWrenchFrame=BaseFrame  EquilibriumPosition=0  EquilibriumPositionUnits=deg  SpringStiffness=0  SpringStiffnessUnits=N*m/deg  DampingCoefficient=0  DampingCoefficientUnits=N*m/(deg/s)  TorqueActuationMode=InputTorque  MotionActuationMode=ComputedMotion  SensePosition=on  SenseVelocity=off  SenseAcceleration=off  SenseTorqueForce=off  PositionTargetSpecify=off  PositionTargetPriority=High  PositionTargetValue=0  PositionTargetValueUnits=deg  VelocityTargetSpecify=off  VelocityTargetPriority=High  VelocityTargetValue=0  VelocityTargetValueUnits=deg/s
  knee : sm_lib/Joints/Revolute Joint  SenseConstraintForce=off  SenseConstraintForceX=off  SenseConstraintForceY=off  SenseConstraintForceZ=off  SenseConstraintTorque=off  SenseConstraintTorqueX=off  SenseConstraintTorqueY=off  SenseConstraintTorqueZ=off  SenseTotalForce=off  SenseTotalForceX=off  SenseTotalForceY=off  SenseTotalForceZ=off  SenseTotalTorque=off  SenseTotalTorqueX=off  SenseTotalTorqueY=off  SenseTotalTorqueZ=off  CompositeWrenchDir=FollowerOnBase  CompositeWrenchFrame=BaseFrame  EquilibriumPosition=0  EquilibriumPositionUnits=deg  SpringStiffness=0  SpringStiffnessUnits=N*m/deg  DampingCoefficient=0  DampingCoefficientUnits=N*m/(deg/s)  TorqueActuationMode=InputTorque  MotionActuationMode=ComputedMotion  SensePosition=on  SenseVelocity=off  SenseAcceleration=off  SenseTorqueForce=off  PositionTargetSpecify=off  PositionTargetPriority=High  PositionTargetValue=0  PositionTargetValueUnits=deg  VelocityTargetSpecify=off  VelocityTargetPriority=High  VelocityTargetValue=0  VelocityTargetValueUnits=deg/s
  lower_leg : sm_lib/Body Elements/Solid  InertiaType=CalculateFromGeometry  Mass=robot.lowerLegWeight  MassUnits=kg  CenterOfMass=[0 0 0]  CenterOfMassUnits=m  MomentsOfInertia=[1 1 1]  MomentsOfInertiaUnits=kg*m^2  ProductsOfInertia=[0 0 0]  ProductsOfInertiaUnits=kg*m^2  BasedOnType=Mass  Density=1000  DensityUnits=kg/m^3  DoExposeReferenceFrame=off  SerializedFrames=<Frames><Frame><Id>Frame1</Id><Value><Name>to_knee</Name><Origin><Source>GeometricFeature</Source><FeatureName>top surface</FeatureName></Origin><PrimaryAxis><DefinedDirection>+X</DefinedDirection><Source>ReferenceFrame</Source><SourceDirection>+X</SourceDirection><FeatureName></FeatureName></PrimaryAxis><SecondaryAxis><DefinedDirection>+Y</DefinedDirection><Source>ReferenceFrame</Source><SourceDirection>-Z</SourceDirection><FeatureName></FeatureName></SecondaryAxis></Value></Frame><Frame><Id>Frame2</Id><Value><Name>to_end</Name><Origin><Source>GeometricFeature</Source><FeatureName>bottom surface</FeatureName></Origin><PrimaryAxis><DefinedDirection>+X</DefinedDirection><Source>ReferenceFrame</Source><SourceDirection>-X</SourceDirection><FeatureName></FeatureName></PrimaryAxis><SecondaryAxis><DefinedDirection>+Y</DefinedDirection><Source>ReferenceFrame</Source><SourceDirection>-Y</SourceDirection><FeatureName></FeatureName></SecondaryAxis></Value></Frame></Frames>  GraphicType=FromGeometry  MarkerShape=Sphere  MarkerSize=10  GraphicVisPropType=SimpleVisualProperties  GraphicDiffuseColor=[0.0 0.4 1.0]  GraphicSpecularColor=[0.5 0.5 0.5 1.0]  GraphicAmbientColor=[0.15 0.15 0.15 1.0]  GraphicEmissiveColor=[0.0 0.0 0.0 1.0]  GraphicShininess=75  GraphicOpacity=1.0  GeometryShape=Cylinder  RectangleSize=[1 1]  RectangleSizeUnits=m  BrickDimensions=[1 1 1]  BrickDimensionUnits=m  CylinderRadius=0.02  CylinderRadiusUnits=m  CylinderLength=robot.lowerLegLength  CylinderLengthUnits=m  SphereRadius=1  SphereRadiusUnits=m  EllipsoidRadii=[1 1 1]  EllipsoidRadiiUnits=m  ExtrusionCrossSection=[1 1; -1 1; -1 -1; 1 -1]  ExtrusionCrossSectionUnits=m  ExtrusionLength=1  ExtrusionLengthUnits=m  PolygonNumSides=3  PolygonOuterRadius=1  PolygonOuterRadiusUnits=m  ExtGeomFileType=STEP  ExtGeomFileUnits=m  RevolutionCrossSection=[1 1; 1 -1; 2 -1; 2 1]  RevolutionCrossSectionUnits=m  RevolutionExtent=Full  RevolutionAngle=180  RevolutionAngleUnits=deg
  q0 : nesl_utility/PS-Simulink Converter  PhysicalDomain=network_engine_domain  SubClassName=ps_output  LeftPortType=input  RightPortType=output  PseudoPeriodic=off  Frequencies=[]  Unit=1  AffineConversion=off
  q1 : nesl_utility/PS-Simulink Converter  PhysicalDomain=network_engine_domain  SubClassName=ps_output  LeftPortType=input  RightPortType=output  PseudoPeriodic=off  Frequencies=[]  Unit=1  AffineConversion=off
  q2 : nesl_utility/PS-Simulink Converter  PhysicalDomain=network_engine_domain  SubClassName=ps_output  LeftPortType=input  RightPortType=output  PseudoPeriodic=off  Frequencies=[]  Unit=1  AffineConversion=off
  shoulder : sm_lib/Joints/Revolute Joint  SenseConstraintForce=off  SenseConstraintForceX=off  SenseConstraintForceY=off  SenseConstraintForceZ=off  SenseConstraintTorque=off  SenseConstraintTorqueX=off  SenseConstraintTorqueY=off  SenseConstraintTorqueZ=off  SenseTotalForce=off  SenseTotalForceX=off  SenseTotalForceY=off  SenseTotalForceZ=off  SenseTotalTorque=off  SenseTotalTorqueX=off  SenseTotalTorqueY=off  SenseTotalTorqueZ=off  CompositeWrenchDir=FollowerOnBase  CompositeWrenchFrame=BaseFrame  EquilibriumPosition=0  EquilibriumPositionUnits=deg  SpringStiffness=0  SpringStiffnessUnits=N*m/deg  DampingCoefficient=0  DampingCoefficientUnits=N*m/(deg/s)  TorqueActuationMode=InputTorque  MotionActuationMode=ComputedMotion  SensePosition=on  SenseVelocity=off  SenseAcceleration=off  SenseTorqueForce=off  PositionTargetSpecify=off  PositionTargetPriority=High  PositionTargetValue=0  PositionTargetValueUnits=deg  VelocityTargetSpecify=off  VelocityTargetPriority=High  VelocityTargetValue=0  VelocityTargetValueUnits=deg/s
  shoulder2hip : sm_lib/Frames and Transforms/Rigid Transform  TranslationMethod=None  TranslationStandardOffset=1.5  TranslationLengthUnit=m  TranslationStandardAxis=+Z  TranslationCartesianOffset=[0 0 0]  TranslationROffset=0  TranslationROffsetUnits=m  TranslationZOffset=0  TranslationZOffsetUnits=m  TranslationThetaOffset=0  TranslationThetaOffsetUnits=deg  RotationMethod=AlignedAxes  RotationAngleUnits=deg  RotationStandardAxis=+X  RotationAngle=90  RotationArbitraryAxis=[0 0 1]  FollAlignAxisA=+X  BaseAlignAxisA=-Z  FollAlignAxisB=+Y  BaseAlignAxisB=+X  RotationSequenceAxes=FollowerAxes  RotationSequence=XYX  RotationSequenceAngles=[0 0 0]  RotationSequenceAnglesUnits=deg  RotationMatrix=[1 0 0; 0 1 0; 0 0 1]
  upper_leg : sm_lib/Body Elements/Solid  InertiaType=CalculateFromGeometry  Mass=robot.upperLegWeight  MassUnits=kg  CenterOfMass=[0 0 0]  CenterOfMassUnits=m  MomentsOfInertia=[1 1 1]  MomentsOfInertiaUnits=kg*m^2  ProductsOfInertia=[0 0 0]  ProductsOfInertiaUnits=kg*m^2  BasedOnType=Mass  Density=1000  DensityUnits=kg/m^3  DoExposeReferenceFrame=off  SerializedFrames=<Frames><Frame><Id>Frame1</Id><Value><Name>to_hip</Name><Origin><Source>GeometricFeature</Source><FeatureName>top surface</FeatureName></Origin><PrimaryAxis><DefinedDirection>+X</DefinedDirection><Source>ReferenceFrame</Source><SourceDirection>+X</SourceDirection><FeatureName></FeatureName></PrimaryAxis><SecondaryAxis><DefinedDirection>+Y</DefinedDirection><Source>ReferenceFrame</Source><SourceDirection>-Z</SourceDirection><FeatureName></FeatureName></SecondaryAxis></Value></Frame><Frame><Id>Frame2</Id><Value><Name>to_knee</Name><Origin><Source>GeometricFeature</Source><FeatureName>bottom curve</FeatureName></Origin><PrimaryAxis><DefinedDirection>+X</DefinedDirection><Source>ReferenceFrame</Source><SourceDirection>+X</SourceDirection><FeatureName></FeatureName></PrimaryAxis><SecondaryAxis><DefinedDirection>+Y</DefinedDirection><Source>ReferenceFrame</Source><SourceDirection>-Z</SourceDirection><FeatureName></FeatureName></SecondaryAxis></Value></Frame></Frames>  GraphicType=FromGeometry  MarkerShape=Sphere  MarkerSize=10  GraphicVisPropType=SimpleVisualProperties  GraphicDiffuseColor=[0.0 0.4 1.0]  GraphicSpecularColor=[0.5 0.5 0.5 1.0]  GraphicAmbientColor=[0.15 0.15 0.15 1.0]  GraphicEmissiveColor=[0.0 0.0 0.0 1.0]  GraphicShininess=75  GraphicOpacity=1.0  GeometryShape=Cylinder  RectangleSize=[1 1]  RectangleSizeUnits=m  BrickDimensions=[1 1 1]  BrickDimensionUnits=m  CylinderRadius=0.02  CylinderRadiusUnits=m  CylinderLength=robot.upperLegLength  CylinderLengthUnits=m  SphereRadius=1  SphereRadiusUnits=m  EllipsoidRadii=[1 1 1]  EllipsoidRadiiUnits=m  ExtrusionCrossSection=[1 1; -1 1; -1 -1; 1 -1]  ExtrusionCrossSectionUnits=m  ExtrusionLength=1  ExtrusionLengthUnits=m  PolygonNumSides=3  PolygonOuterRadius=1  PolygonOuterRadiusUnits=m  ExtGeomFileType=STEP  ExtGeomFileUnits=m  RevolutionCrossSection=[1 1; 1 -1; 2 -1; 2 1]  RevolutionCrossSectionUnits=m  RevolutionExtent=Full  RevolutionAngle=180  RevolutionAngleUnits=deg
  to_body : PMIOPort  Side=Left
  to_ground : PMIOPort  Port=2  Side=Right
  q : Outport
  wires:
  Demux/3 -> Simulink-PS Converter1/1
  Demux/2 -> Simulink-PS Converter/1
  q0/1 -> Mux/1
  q1/1 -> Mux/2
  q2/1 -> Mux/3
  Demux/1 -> Simulink-PS Converter2/1
  tau/1 -> Demux/1
  Mux/1 -> q/1
  connections:
  Simulink-PS Converter/RConn1 -- hip/LConn2
  q0/LConn1 -- shoulder/RConn2
  q2/LConn1 -- knee/RConn2
  knee/LConn1 -- upper_leg/RConn1
  hip/RConn1 -- upper_leg/LConn1
  Shoulder_leg/LConn1 -- shoulder/RConn1
  Simulink-PS Converter1/RConn1 -- knee/LConn2
  q1/LConn1 -- hip/RConn2
  foot/RConn1 -- to_ground/RConn1 -- lower_leg/RConn1
  lower_leg/LConn1 -- knee/RConn1
  shoulder2hip/RConn1 -- hip/LConn1
  Simulink-PS Converter2/RConn1 -- shoulder/LConn2
  Shoulder_leg/RConn1 -- shoulder2hip/LConn1
  to_body/RConn1 -- shoulder/LConn1

== system ForceControl_Quadruped_vmc/FL/Subsystem2 ==
  p : Inport
  v : Inport  Port=2
  Constant : Constant  Value=0
  Constant1 : Constant  Value=0
  Gain : Gain  Gain=10
  Gain1 : Gain
  Sum : Sum  Inputs=|+-
  Sum1 : Sum  Inputs=|+-
  Sum2 : Sum  Inputs=|++
  f : Outport
  wires:
  Sum1/1 -> Gain1/1
  Constant1/1 -> Sum1/1
  Sum/1 -> Gain/1
  Constant/1 -> Sum/1
  Gain1/1 -> Sum2/2
  Gain/1 -> Sum2/1
  v/1 -> Sum1/2
  Sum2/1 -> f/1
  p/1 -> Sum/2

== system ForceControl_Quadruped_vmc/FL/Subsystem3 ==
  p : Inport
  v : Inport  Port=2
  Constant : Constant  Value=-0.6
  Constant1 : Constant  Value=0
  Gain : Gain  Gain=10
  Gain1 : Gain
  Sum : Sum  Inputs=|+-
  Sum1 : Sum  Inputs=|+-
  Sum2 : Sum  Inputs=|++
  f : Outport
  wires:
  Sum1/1 -> Gain1/1
  Constant1/1 -> Sum1/1
  Sum/1 -> Gain/1
  Constant/1 -> Sum/1
  Gain1/1 -> Sum2/2
  Gain/1 -> Sum2/1
  v/1 -> Sum1/2
  Sum2/1 -> f/1
  p/1 -> Sum/2

== system ForceControl_Quadruped_vmc/FL1/Subsystem ==
  p : Inport
  v : Inport  Port=2
  Constant : Constant  Value=0
  Constant1 : Constant  Value=0
  Gain : Gain  Gain=10
  Gain1 : Gain
  Sum : Sum  Inputs=|+-
  Sum1 : Sum  Inputs=|+-
  Sum2 : Sum  Inputs=|++
  f : Outport
  wires:
  Sum1/1 -> Gain1/1
  Constant1/1 -> Sum1/1
  Sum/1 -> Gain/1
  Constant/1 -> Sum/1
  Gain1/1 -> Sum2/2
  Gain/1 -> Sum2/1
  v/1 -> Sum1/2
  Sum2/1 -> f/1
  p/1 -> Sum/2
